simulink model "VV_natural"  (R2018b)
settings: Solver=VariableStepAuto  StartTime=0.0  StopTime=10.0  RelTol=1e-3
settings Model: Creator=kekos  LastModifiedBy=kekos

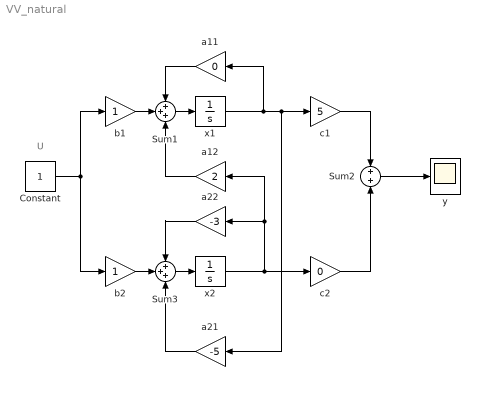
== system VV_natural ==
  note: U
  Constant : Constant
  Sum1 : Sum  Inputs=+++
  Sum2 : Sum
  Sum3 : Sum  Inputs=+++
  a11 : Gain  Gain=0
  a12 : Gain  Gain=2
  a21 : Gain  Gain=-5
  a22 : Gain  Gain=-3
  b1 : Gain
  b2 : Gain
  c1 : Gain  Gain=5
  c2 : Gain  Gain=0
  x1 : Integrator  InitialCondition=0.3
  x2 : Integrator  InitialCondition=0.3
  y : Scope
  wires:
  Constant/1 -> b1/1, b2/1
  b2/1 -> Sum3/2
  x1/1 -> a11/1, a21/1, c1/1
  x2/1 -> a12/1, a22/1, c2/1
  c2/1 -> Sum2/2
  c1/1 -> Sum2/1
  Sum2/1 -> y/1
  Sum1/1 -> x1/1
  a11/1 -> Sum1/1
  b1/1 -> Sum1/2
  a12/1 -> Sum1/3
  Sum3/1 -> x2/1
  a22/1 -> Sum3/1
  a21/1 -> Sum3/3
